simulink model "Mmc_GFL_template"  (R2024b)
settings: Solver=ode23t  StartTime=0.0  StopTime=.3  FixedStep=Ts_Power
undefined symbols (not defined in the file): Ch, Cm, Cmo, Fnom, fs, I_b, Ipp_b, kicir, kiout, kip, kpcir, kpout, kpp, L, L0, Nb_PM, R0, Rdis, Rh, Rm, SCR, SigmaM, Snom, Ts_Power, V_b, VDCm, VDCp, Vnom_AC, Vnom_PM, w_b, Zn
libraries: spsIGBTDiodeLib x48, spsSeriesRLCBranchLib x42, spsVoltageMeasurementLib x17, spsTriangleGeneratorLib x12, spsCurrentMeasurementLib x7, eePwmGeneratorMultilevel x7, slpidlib x6, spsFirstOrderFilterLib x4, spsabctodq0Lib x3, spsGroundLib x2, spsDCVoltageSourceLib x2, spsThreePhaseVIMeasurementLib x2
(part 2 of 3)

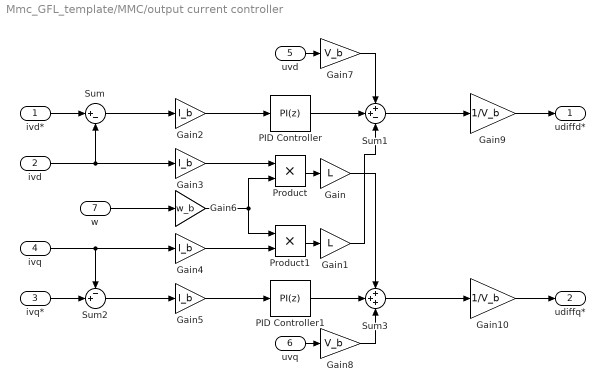
== system Mmc_GFL_template/MMC/output current controller ==
  ivd* : Inport
  ivd : Inport  Port=2
  ivq* : Inport  Port=3
  ivq : Inport  Port=4
  uvd : Inport  Port=5
  uvq : Inport  Port=6
  w : Inport  Port=7
  Gain : Gain  Gain=L
  Gain1 : Gain  Gain=L
  Gain10 : Gain  Gain=1/V_b
  Gain{2..5} (4 alike) : Gain  Gain=I_b
  Gain6 : Gain  Gain=w_b
  Gain7 : Gain  Gain=V_b
  Gain8 : Gain  Gain=V_b
  Gain9 : Gain  Gain=1/V_b
  PID Controller : slpidlib/PID Controller  Controller=PI  Form=Parallel  TimeDomain=Discrete-time  UseExternalTs=off  SampleTime=-1  IntegratorMethod=Forward Euler  FilterMethod=Forward Euler  ControllerParametersSource=internal  P=kpout  I=kiout  UseKiTs=off  D=0  UseExternalDerivativeSource=off  N=100  UseFilter=on  TunerSelectOption=Transfer Function Based (PID Tuner App)  InitialConditionSource=internal  InitialConditionForIntegrator=0  InitialConditionForFilter=0  DifferentiatorICPrevScaledInput=0  ExternalReset=none  TrackingMode=off  Kt=1  LimitOutput=off  SatLimitsSource=internal  UpperSaturationLimit=Vnom_AC  LowerSaturationLimit=-Vnom_AC  LinearizeAsGain=on  AntiWindupMode=clamping  Kb=1  LimitIntegrator=off  UpperIntegratorSaturationLimit=inf  LowerIntegratorSaturationLimit=-inf  POutMin=[]  POutMax=[]  IOutMin=[]  IOutMax=[]  DOutMin=[]  DOutMax=[]  NOutMin=[]  NOutMax=[]  SumOutMin=[]  SumOutMax=[]  SaturationOutMin=[]  SaturationOutMax=[]  PParamMin=[]  PParamMax=[]  IParamMin=[]  IParamMax=[]  DParamMin=[]  DParamMax=[]  NParamMin=[]  NParamMax=[]  KbParamMin=[]  KbParamMax=[]  KtParamMin=[]  KtParamMax=[]  KbOutMin=[]  KbOutMax=[]  KtOutMin=[]  KtOutMax=[]  IntegratorOutMin=[]  IntegratorOutMax=[]  FilterOutMin=[]  FilterOutMax=[]  SumI1OutMin=[]  SumI1OutMax=[]  SumI2OutMin=[]  SumI2OutMax=[]  SumI3OutMin=[]  SumI3OutMax=[]  SumI4OutMin=[]  SumI4OutMax=[]  SumDOutMin=[]  SumDOutMax=[]  DifferentiatorOutMin=[]  DifferentiatorOutMax=[]  FilterDiffOutCoefMin=[]  FilterDiffOutCoefMax=[]  ReciprocalOutMin=[]  ReciprocalOutMax=[]  SumDenOutMin=[]  SumDenOutMax=[]  SumNumOutMin=[]  SumNumOutMax=[]  DivideOutMin=[]  DivideOutMax=[]  UdiffTsProdOutMin=[]  UdiffTsProdOutMax=[]  NTsProdOutMin=[]  NTsProdOutMax=[]  UintegralTsProdOutMin=[]  UintegralTsProdOutMax=[]  UngainTsProdOutMin=[]  UngainTsProdOutMax=[]  ClampingZeroOutDataTypeStr=Inherit: Inherit via back propagation  ClampingZeroOutMin=[]  ClampingZeroOutMax=[]  FilterDenConstantOutDataTypeStr=Inherit: Inherit via back propagation  FilterDenConstantOutMin=[]  FilterDenConstantOutMax=[]  PCopyOutDataTypeStr=Inherit: Inherit via back propagation  PCopyOutMin=[]  PCopyOutMax=[]  NCopyOutDataTypeStr=Inherit: Inherit via back propagation  NCopyOutMin=[]  NCopyOutMax=[]  IntegratorContinuousStateAttributes=''  IntegratorStateMustResolveToSignalObject=off  IntegratorRTWStateStorageClass=Auto  FilterContinuousStateAttributes=''  FilterStateMustResolveToSignalObject=off  FilterRTWStateStorageClass=Auto  ParallelPVariant=InternalParameters  IdealPVariant=Disabled  IVariant=InternalParameters  DVariant=Disabled  IntegratorVariant=Discrete  SatVariant=Disabled  AWVariant=Passthrough  PCopyVariant=Disabled  TRVariant=Disabled  FdbkBlocksVariant=Forward  IdealPFdbkVariant=Disabled  SatFdbkVariant=Disabled  DerivativeFilterVariant=Disabled  NVariant=Disabled  NCopyVariant=Disabled_SignalSpec  FilterICVariant=Disabled  IntegratorICVariant=InternalICs  ExternalResetVariant=Disabled  TRSumVariant=Passthrough  SumFdbkVariant=Disabled  SumVariant=Sum_PI  TsampFilterVariant=InternalTs  TsampNgainVariant=Passthrough  TsampIntegralVariant=Disabled_SignalSpec  ExternalSaturationOutDataTypeStr=Inherit: Same as second input  DerivativeSourceVariant=Disabled  PreIntVariant=InternalPreInt
  PID Controller1 : slpidlib/PID Controller  Controller=PI  Form=Parallel  TimeDomain=Discrete-time  UseExternalTs=off  SampleTime=-1  IntegratorMethod=Forward Euler  FilterMethod=Forward Euler  ControllerParametersSource=internal  P=kpout  I=kiout  UseKiTs=off  D=0  UseExternalDerivativeSource=off  N=100  UseFilter=on  TunerSelectOption=Transfer Function Based (PID Tuner App)  InitialConditionSource=internal  InitialConditionForIntegrator=0  InitialConditionForFilter=0  DifferentiatorICPrevScaledInput=0  ExternalReset=none  TrackingMode=off  Kt=1  LimitOutput=off  SatLimitsSource=internal  UpperSaturationLimit=Vnom_AC  LowerSaturationLimit=-Vnom_AC  LinearizeAsGain=on  AntiWindupMode=clamping  Kb=1  LimitIntegrator=off  UpperIntegratorSaturationLimit=inf  LowerIntegratorSaturationLimit=-inf  POutMin=[]  POutMax=[]  IOutMin=[]  IOutMax=[]  DOutMin=[]  DOutMax=[]  NOutMin=[]  NOutMax=[]  SumOutMin=[]  SumOutMax=[]  SaturationOutMin=[]  SaturationOutMax=[]  PParamMin=[]  PParamMax=[]  IParamMin=[]  IParamMax=[]  DParamMin=[]  DParamMax=[]  NParamMin=[]  NParamMax=[]  KbParamMin=[]  KbParamMax=[]  KtParamMin=[]  KtParamMax=[]  KbOutMin=[]  KbOutMax=[]  KtOutMin=[]  KtOutMax=[]  IntegratorOutMin=[]  IntegratorOutMax=[]  FilterOutMin=[]  FilterOutMax=[]  SumI1OutMin=[]  SumI1OutMax=[]  SumI2OutMin=[]  SumI2OutMax=[]  SumI3OutMin=[]  SumI3OutMax=[]  SumI4OutMin=[]  SumI4OutMax=[]  SumDOutMin=[]  SumDOutMax=[]  DifferentiatorOutMin=[]  DifferentiatorOutMax=[]  FilterDiffOutCoefMin=[]  FilterDiffOutCoefMax=[]  ReciprocalOutMin=[]  ReciprocalOutMax=[]  SumDenOutMin=[]  SumDenOutMax=[]  SumNumOutMin=[]  SumNumOutMax=[]  DivideOutMin=[]  DivideOutMax=[]  UdiffTsProdOutMin=[]  UdiffTsProdOutMax=[]  NTsProdOutMin=[]  NTsProdOutMax=[]  UintegralTsProdOutMin=[]  UintegralTsProdOutMax=[]  UngainTsProdOutMin=[]  UngainTsProdOutMax=[]  ClampingZeroOutDataTypeStr=Inherit: Inherit via back propagation  ClampingZeroOutMin=[]  ClampingZeroOutMax=[]  FilterDenConstantOutDataTypeStr=Inherit: Inherit via back propagation  FilterDenConstantOutMin=[]  FilterDenConstantOutMax=[]  PCopyOutDataTypeStr=Inherit: Inherit via back propagation  PCopyOutMin=[]  PCopyOutMax=[]  NCopyOutDataTypeStr=Inherit: Inherit via back propagation  NCopyOutMin=[]  NCopyOutMax=[]  IntegratorContinuousStateAttributes=''  IntegratorStateMustResolveToSignalObject=off  IntegratorRTWStateStorageClass=Auto  FilterContinuousStateAttributes=''  FilterStateMustResolveToSignalObject=off  FilterRTWStateStorageClass=Auto  ParallelPVariant=InternalParameters  IdealPVariant=Disabled  IVariant=InternalParameters  DVariant=Disabled  IntegratorVariant=Discrete  SatVariant=Disabled  AWVariant=Passthrough  PCopyVariant=Disabled  TRVariant=Disabled  FdbkBlocksVariant=Forward  IdealPFdbkVariant=Disabled  SatFdbkVariant=Disabled  DerivativeFilterVariant=Disabled  NVariant=Disabled  NCopyVariant=Disabled_SignalSpec  FilterICVariant=Disabled  IntegratorICVariant=InternalICs  ExternalResetVariant=Disabled  TRSumVariant=Passthrough  SumFdbkVariant=Disabled  SumVariant=Sum_PI  TsampFilterVariant=InternalTs  TsampNgainVariant=Passthrough  TsampIntegralVariant=Disabled_SignalSpec  ExternalSaturationOutDataTypeStr=Inherit: Same as second input  DerivativeSourceVariant=Disabled  PreIntVariant=InternalPreInt
  Product : Product
  Product1 : Product
  Sum : Sum  Inputs=|+-
  Sum1 : Sum  Inputs=++-
  Sum2 : Sum  Inputs=-+|
  Sum3 : Sum  Inputs=+++
  udiffd* : Outport
  udiffq* : Outport  Port=2
  wires:
  ivd*/1 -> Sum/1
  ivd/1 -> Gain3/1, Sum/2
  Sum/1 -> Gain2/1
  PID Controller/1 -> Sum1/2
  uvd/1 -> Gain7/1
  Sum1/1 -> Gain9/1
  Sum2/1 -> Gain5/1
  PID Controller1/1 -> Sum3/2
  ivq*/1 -> Sum2/2
  ivq/1 -> Sum2/1, Gain4/1
  uvq/1 -> Gain8/1
  Sum3/1 -> Gain10/1
  Product/1 -> Gain/1
  Product1/1 -> Gain1/1
  Gain3/1 -> Product/1
  Gain4/1 -> Product1/2
  Gain5/1 -> PID Controller1/1
  w/1 -> Gain6/1
  Gain6/1 -> Product/2, Product1/1
  Gain9/1 -> udiffd*/1
  Gain10/1 -> udiffq*/1
  Gain7/1 -> Sum1/1
  Gain8/1 -> Sum3/3
  Gain2/1 -> PID Controller/1
  Gain/1 -> Sum3/1
  Gain1/1 -> Sum1/3

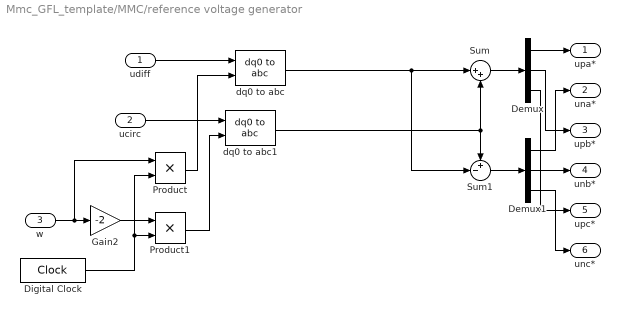
== system Mmc_GFL_template/MMC/reference voltage generator ==
  udiff : Inport
  ucirc : Inport  Port=2
  w : Inport  Port=3
  Demux : Demux  Outputs=3
  Demux1 : Demux  Outputs=3
  Digital Clock : DigitalClock  SampleTime=Ts_Power
  Gain2 : Gain  Gain=-2
  Product : Product
  Product1 : Product
  Sum : Sum  Inputs=|++
  Sum1 : Sum  Inputs=+-|
  dq0 to abc : spsdq0toabcLib/dq0 to abc  Alignment=90 degrees behind phase A axis
  dq0 to abc1 : spsdq0toabcLib/dq0 to abc  Alignment=90 degrees behind phase A axis
  upa* : Outport
  una* : Outport  Port=2
  upb* : Outport  Port=3
  unb* : Outport  Port=4
  upc* : Outport  Port=5
  unc* : Outport  Port=6
  wires:
  Product/1 -> dq0 to abc/2
  udiff/1 -> dq0 to abc/1
  ucirc/1 -> dq0 to abc1/1
  Digital Clock/1 -> Product/2, Product1/2
  Gain2/1 -> Product1/1
  Product1/1 -> dq0 to abc1/2
  w/1 -> Product/1, Gain2/1
  Demux/1 -> upa*/1
  Demux/2 -> upb*/1
  Demux/3 -> upc*/1
  Demux1/1 -> una*/1
  Demux1/2 -> unb*/1
  Demux1/3 -> unc*/1
  Sum/1 -> Demux/1
  Sum1/1 -> Demux1/1
  dq0 to abc1/1 -> Sum/2, Sum1/1
  dq0 to abc/1 -> Sum1/2, Sum/1

== system Mmc_GFL_template/MMC/Full-bridge/HBua1 ==
  gates : Inport
  Ch : spsSeriesRLCBranchLib/Series RLC Branch  LConnTagsString=__new0  RConnTagsString=__new0  BranchType=RC  Resistance=Rh(2,1)  Inductance=1e-3  SetiL0=off  InitialCurrent=0  Capacitance=Ch(2,1)  Setx0=off  InitialVoltage=750  Measurements=None
  Cm : spsSeriesRLCBranchLib/Series RLC Branch  LConnTagsString=__new0  RConnTagsString=__new0  BranchType=RC  Resistance=Rm(2,1)  Inductance=1e-3  SetiL0=off  InitialCurrent=0  Capacitance=Cmo(2,1)  Setx0=on  InitialVoltage=150  Measurements=None
  Demux1 : Demux
  IGBT/Diode{,1..3} (4 alike) : spsIGBTDiodeLib/IGBT//Diode  Ron=Ron  Rs=Rs  Cs=Cs  Measurements=off
  Rdis : spsSeriesRLCBranchLib/Series RLC Branch  LConnTagsString=__new0  RConnTagsString=__new0  BranchType=R  Resistance=Rdis(2,1)  Inductance=1e-3  SetiL0=off  InitialCurrent=0  Capacitance=Cm  Setx0=off  InitialVoltage=750  Measurements=None
  VA : PMIOPort  Side=Left
  VB : PMIOPort  Port=2  Side=Left
  DC+ : PMIOPort  Port=3  Side=Right
  DC- : PMIOPort  Port=4  Side=Right
  wires:
  gates/1 -> Demux1/1
  Demux1/4 -> IGBT/Diode3/1
  Demux1/3 -> IGBT/Diode2/1
  Demux1/2 -> IGBT/Diode1/1
  Demux1/1 -> IGBT/Diode/1
  connections:
  IGBT/Diode3/LConn1 -- VB/RConn1 -- IGBT/Diode2/RConn1
  Ch/LConn1 -- Rdis/LConn1 -- DC+/RConn1 -- IGBT/Diode/LConn1 -- IGBT/Diode2/LConn1 -- Cm/LConn1
  IGBT/Diode/RConn1 -- VA/RConn1 -- IGBT/Diode1/LConn1
  Ch/RConn1 -- DC-/RConn1 -- Rdis/RConn1 -- Cm/RConn1 -- IGBT/Diode3/RConn1 -- IGBT/Diode1/RConn1

== system Mmc_GFL_template/MMC/Full-bridge/HBua2 ==
  gates : Inport
  Ch : spsSeriesRLCBranchLib/Series RLC Branch  LConnTagsString=__new0  RConnTagsString=__new0  BranchType=RC  Resistance=Rh(2,1)  Inductance=1e-3  SetiL0=off  InitialCurrent=0  Capacitance=Ch(2,1)  Setx0=off  InitialVoltage=750  Measurements=None
  Cm : spsSeriesRLCBranchLib/Series RLC Branch  LConnTagsString=__new0  RConnTagsString=__new0  BranchType=RC  Resistance=Rm(2,1)  Inductance=1e-3  SetiL0=off  InitialCurrent=0  Capacitance=Cmo(2,1)  Setx0=on  InitialVoltage=150  Measurements=None
  Demux1 : Demux
  IGBT/Diode{,1..3} (4 alike) : spsIGBTDiodeLib/IGBT//Diode  Ron=Ron  Rs=Rs  Cs=Cs  Measurements=off
  Rdis : spsSeriesRLCBranchLib/Series RLC Branch  LConnTagsString=__new0  RConnTagsString=__new0  BranchType=R  Resistance=Rdis(2,1)  Inductance=1e-3  SetiL0=off  InitialCurrent=0  Capacitance=Cm  Setx0=off  InitialVoltage=750  Measurements=None
  VA : PMIOPort  Side=Left
  VB : PMIOPort  Port=2  Side=Left
  DC+ : PMIOPort  Port=3  Side=Right
  DC- : PMIOPort  Port=4  Side=Right
  wires:
  gates/1 -> Demux1/1
  Demux1/4 -> IGBT/Diode3/1
  Demux1/3 -> IGBT/Diode2/1
  Demux1/2 -> IGBT/Diode1/1
  Demux1/1 -> IGBT/Diode/1
  connections:
  IGBT/Diode3/LConn1 -- VB/RConn1 -- IGBT/Diode2/RConn1
  Ch/LConn1 -- Rdis/LConn1 -- DC+/RConn1 -- IGBT/Diode/LConn1 -- IGBT/Diode2/LConn1 -- Cm/LConn1
  IGBT/Diode/RConn1 -- VA/RConn1 -- IGBT/Diode1/LConn1
  Ch/RConn1 -- DC-/RConn1 -- Rdis/RConn1 -- Cm/RConn1 -- IGBT/Diode3/RConn1 -- IGBT/Diode1/RConn1

== system Mmc_GFL_template/MMC/Full-bridge 1/HBua1 ==
  gates : Inport
  Ch : spsSeriesRLCBranchLib/Series RLC Branch  LConnTagsString=__new0  RConnTagsString=__new0  BranchType=RC  Resistance=Rh(2,1)  Inductance=1e-3  SetiL0=off  InitialCurrent=0  Capacitance=Ch(2,1)  Setx0=off  InitialVoltage=750  Measurements=None
  Cm : spsSeriesRLCBranchLib/Series RLC Branch  LConnTagsString=__new0  RConnTagsString=__new0  BranchType=RC  Resistance=Rm(2,1)  Inductance=1e-3  SetiL0=off  InitialCurrent=0  Capacitance=Cmo(2,1)  Setx0=on  InitialVoltage=150  Measurements=None
  Demux1 : Demux
  IGBT/Diode{,1..3} (4 alike) : spsIGBTDiodeLib/IGBT//Diode  Ron=Ron  Rs=Rs  Cs=Cs  Measurements=off
  Rdis : spsSeriesRLCBranchLib/Series RLC Branch  LConnTagsString=__new0  RConnTagsString=__new0  BranchType=R  Resistance=Rdis(2,1)  Inductance=1e-3  SetiL0=off  InitialCurrent=0  Capacitance=Cm  Setx0=off  InitialVoltage=750  Measurements=None
  VA : PMIOPort  Side=Left
  VB : PMIOPort  Port=2  Side=Left
  DC+ : PMIOPort  Port=3  Side=Right
  DC- : PMIOPort  Port=4  Side=Right
  wires:
  gates/1 -> Demux1/1
  Demux1/4 -> IGBT/Diode3/1
  Demux1/3 -> IGBT/Diode2/1
  Demux1/2 -> IGBT/Diode1/1
  Demux1/1 -> IGBT/Diode/1
  connections:
  IGBT/Diode3/LConn1 -- VB/RConn1 -- IGBT/Diode2/RConn1
  Ch/LConn1 -- Rdis/LConn1 -- DC+/RConn1 -- IGBT/Diode/LConn1 -- IGBT/Diode2/LConn1 -- Cm/LConn1
  IGBT/Diode/RConn1 -- VA/RConn1 -- IGBT/Diode1/LConn1
  Ch/RConn1 -- DC-/RConn1 -- Rdis/RConn1 -- Cm/RConn1 -- IGBT/Diode3/RConn1 -- IGBT/Diode1/RConn1

== system Mmc_GFL_template/MMC/Full-bridge 1/HBua2 ==
  gates : Inport
  Ch : spsSeriesRLCBranchLib/Series RLC Branch  LConnTagsString=__new0  RConnTagsString=__new0  BranchType=RC  Resistance=Rh(2,1)  Inductance=1e-3  SetiL0=off  InitialCurrent=0  Capacitance=Ch(2,1)  Setx0=off  InitialVoltage=750  Measurements=None
  Cm : spsSeriesRLCBranchLib/Series RLC Branch  LConnTagsString=__new0  RConnTagsString=__new0  BranchType=RC  Resistance=Rm(2,1)  Inductance=1e-3  SetiL0=off  InitialCurrent=0  Capacitance=Cmo(2,1)  Setx0=on  InitialVoltage=150  Measurements=None
  Demux1 : Demux
  IGBT/Diode{,1..3} (4 alike) : spsIGBTDiodeLib/IGBT//Diode  Ron=Ron  Rs=Rs  Cs=Cs  Measurements=off
  Rdis : spsSeriesRLCBranchLib/Series RLC Branch  LConnTagsString=__new0  RConnTagsString=__new0  BranchType=R  Resistance=Rdis(2,1)  Inductance=1e-3  SetiL0=off  InitialCurrent=0  Capacitance=Cm  Setx0=off  InitialVoltage=750  Measurements=None
  VA : PMIOPort  Side=Left
  VB : PMIOPort  Port=2  Side=Left
  DC+ : PMIOPort  Port=3  Side=Right
  DC- : PMIOPort  Port=4  Side=Right
  wires:
  gates/1 -> Demux1/1
  Demux1/4 -> IGBT/Diode3/1
  Demux1/3 -> IGBT/Diode2/1
  Demux1/2 -> IGBT/Diode1/1
  Demux1/1 -> IGBT/Diode/1
  connections:
  IGBT/Diode3/LConn1 -- VB/RConn1 -- IGBT/Diode2/RConn1
  Ch/LConn1 -- Rdis/LConn1 -- DC+/RConn1 -- IGBT/Diode/LConn1 -- IGBT/Diode2/LConn1 -- Cm/LConn1
  IGBT/Diode/RConn1 -- VA/RConn1 -- IGBT/Diode1/LConn1
  Ch/RConn1 -- DC-/RConn1 -- Rdis/RConn1 -- Cm/RConn1 -- IGBT/Diode3/RConn1 -- IGBT/Diode1/RConn1

== system Mmc_GFL_template/MMC/Full-bridge 2/HBua1 ==
  gates : Inport
  Ch : spsSeriesRLCBranchLib/Series RLC Branch  LConnTagsString=__new0  RConnTagsString=__new0  BranchType=RC  Resistance=Rh(2,1)  Inductance=1e-3  SetiL0=off  InitialCurrent=0  Capacitance=Ch(2,1)  Setx0=off  InitialVoltage=750  Measurements=None
  Cm : spsSeriesRLCBranchLib/Series RLC Branch  LConnTagsString=__new0  RConnTagsString=__new0  BranchType=RC  Resistance=Rm(2,1)  Inductance=1e-3  SetiL0=off  InitialCurrent=0  Capacitance=Cmo(2,1)  Setx0=on  InitialVoltage=150  Measurements=None
  Demux1 : Demux
  IGBT/Diode{,1..3} (4 alike) : spsIGBTDiodeLib/IGBT//Diode  Ron=Ron  Rs=Rs  Cs=Cs  Measurements=off
  Rdis : spsSeriesRLCBranchLib/Series RLC Branch  LConnTagsString=__new0  RConnTagsString=__new0  BranchType=R  Resistance=Rdis(2,1)  Inductance=1e-3  SetiL0=off  InitialCurrent=0  Capacitance=Cm  Setx0=off  InitialVoltage=750  Measurements=None
  VA : PMIOPort  Side=Left
  VB : PMIOPort  Port=2  Side=Left
  DC+ : PMIOPort  Port=3  Side=Right
  DC- : PMIOPort  Port=4  Side=Right
  wires:
  gates/1 -> Demux1/1
  Demux1/4 -> IGBT/Diode3/1
  Demux1/3 -> IGBT/Diode2/1
  Demux1/2 -> IGBT/Diode1/1
  Demux1/1 -> IGBT/Diode/1
  connections:
  IGBT/Diode3/LConn1 -- VB/RConn1 -- IGBT/Diode2/RConn1
  Ch/LConn1 -- Rdis/LConn1 -- DC+/RConn1 -- IGBT/Diode/LConn1 -- IGBT/Diode2/LConn1 -- Cm/LConn1
  IGBT/Diode/RConn1 -- VA/RConn1 -- IGBT/Diode1/LConn1
  Ch/RConn1 -- DC-/RConn1 -- Rdis/RConn1 -- Cm/RConn1 -- IGBT/Diode3/RConn1 -- IGBT/Diode1/RConn1

== system Mmc_GFL_template/MMC/Full-bridge 2/HBua2 ==
  gates : Inport
  Ch : spsSeriesRLCBranchLib/Series RLC Branch  LConnTagsString=__new0  RConnTagsString=__new0  BranchType=RC  Resistance=Rh(2,1)  Inductance=1e-3  SetiL0=off  InitialCurrent=0  Capacitance=Ch(2,1)  Setx0=off  InitialVoltage=750  Measurements=None
  Cm : spsSeriesRLCBranchLib/Series RLC Branch  LConnTagsString=__new0  RConnTagsString=__new0  BranchType=RC  Resistance=Rm(2,1)  Inductance=1e-3  SetiL0=off  InitialCurrent=0  Capacitance=Cmo(2,1)  Setx0=on  InitialVoltage=150  Measurements=None
  Demux1 : Demux
  IGBT/Diode{,1..3} (4 alike) : spsIGBTDiodeLib/IGBT//Diode  Ron=Ron  Rs=Rs  Cs=Cs  Measurements=off
  Rdis : spsSeriesRLCBranchLib/Series RLC Branch  LConnTagsString=__new0  RConnTagsString=__new0  BranchType=R  Resistance=Rdis(2,1)  Inductance=1e-3  SetiL0=off  InitialCurrent=0  Capacitance=Cm  Setx0=off  InitialVoltage=750  Measurements=None
  VA : PMIOPort  Side=Left
  VB : PMIOPort  Port=2  Side=Left
  DC+ : PMIOPort  Port=3  Side=Right
  DC- : PMIOPort  Port=4  Side=Right
  wires:
  gates/1 -> Demux1/1
  Demux1/4 -> IGBT/Diode3/1
  Demux1/3 -> IGBT/Diode2/1
  Demux1/2 -> IGBT/Diode1/1
  Demux1/1 -> IGBT/Diode/1
  connections:
  IGBT/Diode3/LConn1 -- VB/RConn1 -- IGBT/Diode2/RConn1
  Ch/LConn1 -- Rdis/LConn1 -- DC+/RConn1 -- IGBT/Diode/LConn1 -- IGBT/Diode2/LConn1 -- Cm/LConn1
  IGBT/Diode/RConn1 -- VA/RConn1 -- IGBT/Diode1/LConn1
  Ch/RConn1 -- DC-/RConn1 -- Rdis/RConn1 -- Cm/RConn1 -- IGBT/Diode3/RConn1 -- IGBT/Diode1/RConn1

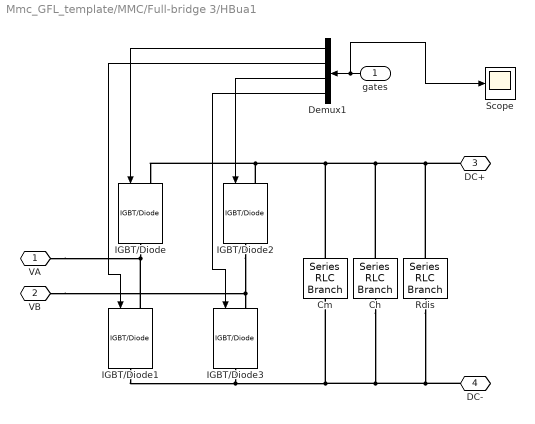
== system Mmc_GFL_template/MMC/Full-bridge 3/HBua1 ==
  gates : Inport
  Ch : spsSeriesRLCBranchLib/Series RLC Branch  LConnTagsString=__new0  RConnTagsString=__new0  BranchType=RC  Resistance=Rh(2,1)  Inductance=1e-3  SetiL0=off  InitialCurrent=0  Capacitance=Ch(2,1)  Setx0=off  InitialVoltage=750  Measurements=None
  Cm : spsSeriesRLCBranchLib/Series RLC Branch  LConnTagsString=__new0  RConnTagsString=__new0  BranchType=RC  Resistance=Rm(2,1)  Inductance=1e-3  SetiL0=off  InitialCurrent=0  Capacitance=Cmo(2,1)  Setx0=on  InitialVoltage=150  Measurements=None
  Demux1 : Demux
  IGBT/Diode{,1..3} (4 alike) : spsIGBTDiodeLib/IGBT//Diode  Ron=Ron  Rs=Rs  Cs=Cs  Measurements=off
  Rdis : spsSeriesRLCBranchLib/Series RLC Branch  LConnTagsString=__new0  RConnTagsString=__new0  BranchType=R  Resistance=Rdis(2,1)  Inductance=1e-3  SetiL0=off  InitialCurrent=0  Capacitance=Cm  Setx0=off  InitialVoltage=750  Measurements=None
  Scope : Scope
  VA : PMIOPort  Side=Left
  VB : PMIOPort  Port=2  Side=Left
  DC+ : PMIOPort  Port=3  Side=Right
  DC- : PMIOPort  Port=4  Side=Right
  wires:
  gates/1 -> Scope/1, Demux1/1
  Demux1/4 -> IGBT/Diode3/1
  Demux1/3 -> IGBT/Diode2/1
  Demux1/2 -> IGBT/Diode1/1
  Demux1/1 -> IGBT/Diode/1
  connections:
  IGBT/Diode3/LConn1 -- VB/RConn1 -- IGBT/Diode2/RConn1
  Ch/LConn1 -- Rdis/LConn1 -- DC+/RConn1 -- IGBT/Diode/LConn1 -- IGBT/Diode2/LConn1 -- Cm/LConn1
  IGBT/Diode/RConn1 -- VA/RConn1 -- IGBT/Diode1/LConn1
  Ch/RConn1 -- DC-/RConn1 -- Rdis/RConn1 -- Cm/RConn1 -- IGBT/Diode3/RConn1 -- IGBT/Diode1/RConn1

== system Mmc_GFL_template/MMC/Full-bridge 3/HBua2 ==
  gates : Inport
  Ch : spsSeriesRLCBranchLib/Series RLC Branch  LConnTagsString=__new0  RConnTagsString=__new0  BranchType=RC  Resistance=Rh(2,1)  Inductance=1e-3  SetiL0=off  InitialCurrent=0  Capacitance=Ch(2,1)  Setx0=off  InitialVoltage=750  Measurements=None
  Cm : spsSeriesRLCBranchLib/Series RLC Branch  LConnTagsString=__new0  RConnTagsString=__new0  BranchType=RC  Resistance=Rm(2,1)  Inductance=1e-3  SetiL0=off  InitialCurrent=0  Capacitance=Cmo(2,1)  Setx0=on  InitialVoltage=150  Measurements=None
  Demux1 : Demux
  IGBT/Diode{,1..3} (4 alike) : spsIGBTDiodeLib/IGBT//Diode  Ron=Ron  Rs=Rs  Cs=Cs  Measurements=off
  Rdis : spsSeriesRLCBranchLib/Series RLC Branch  LConnTagsString=__new0  RConnTagsString=__new0  BranchType=R  Resistance=Rdis(2,1)  Inductance=1e-3  SetiL0=off  InitialCurrent=0  Capacitance=Cm  Setx0=off  InitialVoltage=750  Measurements=None
  VA : PMIOPort  Side=Left
  VB : PMIOPort  Port=2  Side=Left
  DC+ : PMIOPort  Port=3  Side=Right
  DC- : PMIOPort  Port=4  Side=Right
  wires:
  gates/1 -> Demux1/1
  Demux1/4 -> IGBT/Diode3/1
  Demux1/3 -> IGBT/Diode2/1
  Demux1/2 -> IGBT/Diode1/1
  Demux1/1 -> IGBT/Diode/1
  connections:
  IGBT/Diode3/LConn1 -- VB/RConn1 -- IGBT/Diode2/RConn1
  Ch/LConn1 -- Rdis/LConn1 -- DC+/RConn1 -- IGBT/Diode/LConn1 -- IGBT/Diode2/LConn1 -- Cm/LConn1
  IGBT/Diode/RConn1 -- VA/RConn1 -- IGBT/Diode1/LConn1
  Ch/RConn1 -- DC-/RConn1 -- Rdis/RConn1 -- Cm/RConn1 -- IGBT/Diode3/RConn1 -- IGBT/Diode1/RConn1

== system Mmc_GFL_template/MMC/Full-bridge 4/HBua1 ==
  gates : Inport
  Ch : spsSeriesRLCBranchLib/Series RLC Branch  LConnTagsString=__new0  RConnTagsString=__new0  BranchType=RC  Resistance=Rh(2,1)  Inductance=1e-3  SetiL0=off  InitialCurrent=0  Capacitance=Ch(2,1)  Setx0=off  InitialVoltage=750  Measurements=None
  Cm : spsSeriesRLCBranchLib/Series RLC Branch  LConnTagsString=__new0  RConnTagsString=__new0  BranchType=RC  Resistance=Rm(2,1)  Inductance=1e-3  SetiL0=off  InitialCurrent=0  Capacitance=Cmo(2,1)  Setx0=on  InitialVoltage=150  Measurements=None
  Demux1 : Demux
  IGBT/Diode{,1..3} (4 alike) : spsIGBTDiodeLib/IGBT//Diode  Ron=Ron  Rs=Rs  Cs=Cs  Measurements=off
  Rdis : spsSeriesRLCBranchLib/Series RLC Branch  LConnTagsString=__new0  RConnTagsString=__new0  BranchType=R  Resistance=Rdis(2,1)  Inductance=1e-3  SetiL0=off  InitialCurrent=0  Capacitance=Cm  Setx0=off  InitialVoltage=750  Measurements=None
  VA : PMIOPort  Side=Left
  VB : PMIOPort  Port=2  Side=Left
  DC+ : PMIOPort  Port=3  Side=Right
  DC- : PMIOPort  Port=4  Side=Right
  wires:
  gates/1 -> Demux1/1
  Demux1/4 -> IGBT/Diode3/1
  Demux1/3 -> IGBT/Diode2/1
  Demux1/2 -> IGBT/Diode1/1
  Demux1/1 -> IGBT/Diode/1
  connections:
  IGBT/Diode3/LConn1 -- VB/RConn1 -- IGBT/Diode2/RConn1
  Ch/LConn1 -- Rdis/LConn1 -- DC+/RConn1 -- IGBT/Diode/LConn1 -- IGBT/Diode2/LConn1 -- Cm/LConn1
  IGBT/Diode/RConn1 -- VA/RConn1 -- IGBT/Diode1/LConn1
  Ch/RConn1 -- DC-/RConn1 -- Rdis/RConn1 -- Cm/RConn1 -- IGBT/Diode3/RConn1 -- IGBT/Diode1/RConn1

== system Mmc_GFL_template/MMC/Full-bridge 4/HBua2 ==
  gates : Inport
  Ch : spsSeriesRLCBranchLib/Series RLC Branch  LConnTagsString=__new0  RConnTagsString=__new0  BranchType=RC  Resistance=Rh(2,1)  Inductance=1e-3  SetiL0=off  InitialCurrent=0  Capacitance=Ch(2,1)  Setx0=off  InitialVoltage=750  Measurements=None
  Cm : spsSeriesRLCBranchLib/Series RLC Branch  LConnTagsString=__new0  RConnTagsString=__new0  BranchType=RC  Resistance=Rm(2,1)  Inductance=1e-3  SetiL0=off  InitialCurrent=0  Capacitance=Cmo(2,1)  Setx0=on  InitialVoltage=150  Measurements=None
  Demux1 : Demux
  IGBT/Diode{,1..3} (4 alike) : spsIGBTDiodeLib/IGBT//Diode  Ron=Ron  Rs=Rs  Cs=Cs  Measurements=off
  Rdis : spsSeriesRLCBranchLib/Series RLC Branch  LConnTagsString=__new0  RConnTagsString=__new0  BranchType=R  Resistance=Rdis(2,1)  Inductance=1e-3  SetiL0=off  InitialCurrent=0  Capacitance=Cm  Setx0=off  InitialVoltage=750  Measurements=None
  VA : PMIOPort  Side=Left
  VB : PMIOPort  Port=2  Side=Left
  DC+ : PMIOPort  Port=3  Side=Right
  DC- : PMIOPort  Port=4  Side=Right
  wires:
  gates/1 -> Demux1/1
  Demux1/4 -> IGBT/Diode3/1
  Demux1/3 -> IGBT/Diode2/1
  Demux1/2 -> IGBT/Diode1/1
  Demux1/1 -> IGBT/Diode/1
  connections:
  IGBT/Diode3/LConn1 -- VB/RConn1 -- IGBT/Diode2/RConn1
  Ch/LConn1 -- Rdis/LConn1 -- DC+/RConn1 -- IGBT/Diode/LConn1 -- IGBT/Diode2/LConn1 -- Cm/LConn1
  IGBT/Diode/RConn1 -- VA/RConn1 -- IGBT/Diode1/LConn1
  Ch/RConn1 -- DC-/RConn1 -- Rdis/RConn1 -- Cm/RConn1 -- IGBT/Diode3/RConn1 -- IGBT/Diode1/RConn1

== system Mmc_GFL_template/MMC/Full-bridge 5/HBua1 ==
  gates : Inport
  Ch : spsSeriesRLCBranchLib/Series RLC Branch  LConnTagsString=__new0  RConnTagsString=__new0  BranchType=RC  Resistance=Rh(2,1)  Inductance=1e-3  SetiL0=off  InitialCurrent=0  Capacitance=Ch(2,1)  Setx0=off  InitialVoltage=750  Measurements=None
  Cm : spsSeriesRLCBranchLib/Series RLC Branch  LConnTagsString=__new0  RConnTagsString=__new0  BranchType=RC  Resistance=Rm(2,1)  Inductance=1e-3  SetiL0=off  InitialCurrent=0  Capacitance=Cmo(2,1)  Setx0=on  InitialVoltage=150  Measurements=None
  Demux1 : Demux
  IGBT/Diode{,1..3} (4 alike) : spsIGBTDiodeLib/IGBT//Diode  Ron=Ron  Rs=Rs  Cs=Cs  Measurements=off
  Rdis : spsSeriesRLCBranchLib/Series RLC Branch  LConnTagsString=__new0  RConnTagsString=__new0  BranchType=R  Resistance=Rdis(2,1)  Inductance=1e-3  SetiL0=off  InitialCurrent=0  Capacitance=Cm  Setx0=off  InitialVoltage=750  Measurements=None
  VA : PMIOPort  Side=Left
  VB : PMIOPort  Port=2  Side=Left
  DC+ : PMIOPort  Port=3  Side=Right
  DC- : PMIOPort  Port=4  Side=Right
  wires:
  gates/1 -> Demux1/1
  Demux1/4 -> IGBT/Diode3/1
  Demux1/3 -> IGBT/Diode2/1
  Demux1/2 -> IGBT/Diode1/1
  Demux1/1 -> IGBT/Diode/1
  connections:
  IGBT/Diode3/LConn1 -- VB/RConn1 -- IGBT/Diode2/RConn1
  Ch/LConn1 -- Rdis/LConn1 -- DC+/RConn1 -- IGBT/Diode/LConn1 -- IGBT/Diode2/LConn1 -- Cm/LConn1
  IGBT/Diode/RConn1 -- VA/RConn1 -- IGBT/Diode1/LConn1
  Ch/RConn1 -- DC-/RConn1 -- Rdis/RConn1 -- Cm/RConn1 -- IGBT/Diode3/RConn1 -- IGBT/Diode1/RConn1

== system Mmc_GFL_template/MMC/Full-bridge 5/HBua2 ==
  gates : Inport
  Ch : spsSeriesRLCBranchLib/Series RLC Branch  LConnTagsString=__new0  RConnTagsString=__new0  BranchType=RC  Resistance=Rh(2,1)  Inductance=1e-3  SetiL0=off  InitialCurrent=0  Capacitance=Ch(2,1)  Setx0=off  InitialVoltage=750  Measurements=None
  Cm : spsSeriesRLCBranchLib/Series RLC Branch  LConnTagsString=__new0  RConnTagsString=__new0  BranchType=RC  Resistance=Rm(2,1)  Inductance=1e-3  SetiL0=off  InitialCurrent=0  Capacitance=Cmo(2,1)  Setx0=on  InitialVoltage=150  Measurements=None
  Demux1 : Demux
  IGBT/Diode{,1..3} (4 alike) : spsIGBTDiodeLib/IGBT//Diode  Ron=Ron  Rs=Rs  Cs=Cs  Measurements=off
  Rdis : spsSeriesRLCBranchLib/Series RLC Branch  LConnTagsString=__new0  RConnTagsString=__new0  BranchType=R  Resistance=Rdis(2,1)  Inductance=1e-3  SetiL0=off  InitialCurrent=0  Capacitance=Cm  Setx0=off  InitialVoltage=750  Measurements=None
  VA : PMIOPort  Side=Left
  VB : PMIOPort  Port=2  Side=Left
  DC+ : PMIOPort  Port=3  Side=Right
  DC- : PMIOPort  Port=4  Side=Right
  wires:
  gates/1 -> Demux1/1
  Demux1/4 -> IGBT/Diode3/1
  Demux1/3 -> IGBT/Diode2/1
  Demux1/2 -> IGBT/Diode1/1
  Demux1/1 -> IGBT/Diode/1
  connections:
  IGBT/Diode3/LConn1 -- VB/RConn1 -- IGBT/Diode2/RConn1
  Ch/LConn1 -- Rdis/LConn1 -- DC+/RConn1 -- IGBT/Diode/LConn1 -- IGBT/Diode2/LConn1 -- Cm/LConn1
  IGBT/Diode/RConn1 -- VA/RConn1 -- IGBT/Diode1/LConn1
  Ch/RConn1 -- DC-/RConn1 -- Rdis/RConn1 -- Cm/RConn1 -- IGBT/Diode3/RConn1 -- IGBT/Diode1/RConn1

== system Mmc_GFL_template/MMC/PS-PWM/PS-PWM lower a ==
  ref : Inport
  Gain : Gain  Gain=70
  Gain1 : Gain  Gain=70
  Logical Operator : Logic  Operator=NOT  AllPortsSameDT=off  OutDataTypeStr=boolean
  Logical Operator1 : Logic  Operator=NOT  AllPortsSameDT=off  OutDataTypeStr=boolean
  Mux : Mux
  Relational Operator : RelationalOperator  OutDataTypeStr=boolean  RndMeth=Simplest  InputSameDT=off
  Relational Operator1 : RelationalOperator  OutDataTypeStr=boolean  RndMeth=Simplest  InputSameDT=off
  Triangle Generator : spsTriangleGeneratorLib/Triangle Generator  Freq=1e3  Phase=0  Ts=Ts_Power
  Triangle Generator1 : spsTriangleGeneratorLib/Triangle Generator  Freq=1e3  Phase=pi/(4)  Ts=Ts_Power
  Ppa : Outport
  wires:
  Logical Operator/1 -> Mux/2
  ref/1 -> Relational Operator1/1, Relational Operator/1
  Relational Operator/1 -> Mux/1, Logical Operator/1
  Relational Operator1/1 -> Logical Operator1/1, Mux/3
  Triangle Generator/1 -> Gain/1
  Triangle Generator1/1 -> Gain1/1
  Mux/1 -> Ppa/1
  Logical Operator1/1 -> Mux/4
  Gain1/1 -> Relational Operator1/2
  Gain/1 -> Relational Operator/2

== system Mmc_GFL_template/MMC/PS-PWM/PS-PWM lower b ==
  ref : Inport
  Gain : Gain  Gain=70
  Gain1 : Gain  Gain=70
  Logical Operator : Logic  Operator=NOT  AllPortsSameDT=off  OutDataTypeStr=boolean
  Logical Operator1 : Logic  Operator=NOT  AllPortsSameDT=off  OutDataTypeStr=boolean
  Mux : Mux
  Relational Operator : RelationalOperator  OutDataTypeStr=boolean  RndMeth=Simplest  InputSameDT=off
  Relational Operator1 : RelationalOperator  OutDataTypeStr=boolean  RndMeth=Simplest  InputSameDT=off
  Triangle Generator : spsTriangleGeneratorLib/Triangle Generator  Freq=1e3  Phase=0  Ts=Ts_Power
  Triangle Generator1 : spsTriangleGeneratorLib/Triangle Generator  Freq=1e3  Phase=pi/(4)  Ts=Ts_Power
  Ppa : Outport
  wires:
  Logical Operator/1 -> Mux/2
  ref/1 -> Relational Operator1/1, Relational Operator/1
  Relational Operator/1 -> Mux/1, Logical Operator/1
  Relational Operator1/1 -> Logical Operator1/1, Mux/3
  Triangle Generator/1 -> Gain/1
  Triangle Generator1/1 -> Gain1/1
  Mux/1 -> Ppa/1
  Logical Operator1/1 -> Mux/4
  Gain/1 -> Relational Operator/2
  Gain1/1 -> Relational Operator1/2

== system Mmc_GFL_template/MMC/PS-PWM/PS-PWM lower c ==
  ref : Inport
  Gain : Gain  Gain=70
  Gain1 : Gain  Gain=70
  Logical Operator : Logic  Operator=NOT  AllPortsSameDT=off  OutDataTypeStr=boolean
  Logical Operator1 : Logic  Operator=NOT  AllPortsSameDT=off  OutDataTypeStr=boolean
  Mux : Mux
  Relational Operator : RelationalOperator  OutDataTypeStr=boolean  RndMeth=Simplest  InputSameDT=off
  Relational Operator1 : RelationalOperator  OutDataTypeStr=boolean  RndMeth=Simplest  InputSameDT=off
  Triangle Generator : spsTriangleGeneratorLib/Triangle Generator  Freq=1e3  Phase=0  Ts=Ts_Power
  Triangle Generator1 : spsTriangleGeneratorLib/Triangle Generator  Freq=1e3  Phase=pi/(4)  Ts=Ts_Power
  Ppa : Outport
  wires:
  Logical Operator/1 -> Mux/2
  ref/1 -> Relational Operator1/1, Relational Operator/1
  Relational Operator/1 -> Mux/1, Logical Operator/1
  Relational Operator1/1 -> Logical Operator1/1, Mux/3
  Triangle Generator/1 -> Gain/1
  Triangle Generator1/1 -> Gain1/1
  Mux/1 -> Ppa/1
  Logical Operator1/1 -> Mux/4
  Gain/1 -> Relational Operator/2
  Gain1/1 -> Relational Operator1/2

== system Mmc_GFL_template/MMC/PS-PWM/PS-PWM upper a ==
  ref : Inport
  Gain : Gain  Gain=70
  Gain1 : Gain  Gain=70
  Logical Operator : Logic  Operator=NOT  AllPortsSameDT=off  OutDataTypeStr=boolean
  Logical Operator1 : Logic  Operator=NOT  AllPortsSameDT=off  OutDataTypeStr=boolean
  Mux : Mux
  Relational Operator : RelationalOperator  OutDataTypeStr=boolean  RndMeth=Simplest  InputSameDT=off
  Relational Operator1 : RelationalOperator  OutDataTypeStr=boolean  RndMeth=Simplest  InputSameDT=off
  Scope : Scope
  Triangle Generator : spsTriangleGeneratorLib/Triangle Generator  Freq=1e3  Phase=0  Ts=Ts_Power
  Triangle Generator1 : spsTriangleGeneratorLib/Triangle Generator  Freq=1e3  Phase=pi/(4)  Ts=Ts_Power
  Ppa : Outport
  wires:
  Triangle Generator1/1 -> Gain1/1
  Triangle Generator/1 -> Gain/1
  ref/1 -> Scope/1, Relational Operator1/1, Relational Operator/1
  Mux/1 -> Ppa/1
  Relational Operator/1 -> Mux/1, Logical Operator/1
  Relational Operator1/1 -> Logical Operator1/1, Mux/3
  Logical Operator/1 -> Mux/2
  Logical Operator1/1 -> Mux/4
  Gain/1 -> Relational Operator/2
  Gain1/1 -> Relational Operator1/2

== system Mmc_GFL_template/MMC/PS-PWM/PS-PWM upper b ==
  ref : Inport
  Gain : Gain  Gain=70
  Gain1 : Gain  Gain=70
  Logical Operator : Logic  Operator=NOT  AllPortsSameDT=off  OutDataTypeStr=boolean
  Logical Operator1 : Logic  Operator=NOT  AllPortsSameDT=off  OutDataTypeStr=boolean
  Mux : Mux
  Relational Operator : RelationalOperator  OutDataTypeStr=boolean  RndMeth=Simplest  InputSameDT=off
  Relational Operator1 : RelationalOperator  OutDataTypeStr=boolean  RndMeth=Simplest  InputSameDT=off
  Triangle Generator : spsTriangleGeneratorLib/Triangle Generator  Freq=1e3  Phase=0  Ts=Ts_Power
  Triangle Generator1 : spsTriangleGeneratorLib/Triangle Generator  Freq=1e3  Phase=pi/(4)  Ts=Ts_Power
  Ppa : Outport
  wires:
  Triangle Generator1/1 -> Gain1/1
  Triangle Generator/1 -> Gain/1
  ref/1 -> Relational Operator1/1, Relational Operator/1
  Mux/1 -> Ppa/1
  Relational Operator/1 -> Mux/1, Logical Operator/1
  Relational Operator1/1 -> Logical Operator1/1, Mux/3
  Logical Operator/1 -> Mux/2
  Logical Operator1/1 -> Mux/4
  Gain/1 -> Relational Operator/2
  Gain1/1 -> Relational Operator1/2

== system Mmc_GFL_template/MMC/PS-PWM/PS-PWM upper c ==
  ref : Inport
  Gain : Gain  Gain=70
  Gain1 : Gain  Gain=70
  Logical Operator : Logic  Operator=NOT  AllPortsSameDT=off  OutDataTypeStr=boolean
  Logical Operator1 : Logic  Operator=NOT  AllPortsSameDT=off  OutDataTypeStr=boolean
  Mux : Mux
  Relational Operator : RelationalOperator  OutDataTypeStr=boolean  RndMeth=Simplest  InputSameDT=off
  Relational Operator1 : RelationalOperator  OutDataTypeStr=boolean  RndMeth=Simplest  InputSameDT=off
  Triangle Generator : spsTriangleGeneratorLib/Triangle Generator  Freq=1e3  Phase=0  Ts=Ts_Power
  Triangle Generator1 : spsTriangleGeneratorLib/Triangle Generator  Freq=1e3  Phase=pi/(4)  Ts=Ts_Power
  Ppa : Outport
  wires:
  Triangle Generator1/1 -> Gain1/1
  Triangle Generator/1 -> Gain/1
  ref/1 -> Relational Operator1/1, Relational Operator/1
  Mux/1 -> Ppa/1
  Relational Operator/1 -> Mux/1, Logical Operator/1
  Relational Operator1/1 -> Logical Operator1/1, Mux/3
  Logical Operator/1 -> Mux/2
  Logical Operator1/1 -> Mux/4
  Gain/1 -> Relational Operator/2
  Gain1/1 -> Relational Operator1/2

== system Mmc_GFL_template/MMC/modulation/Sorting na ==
  note: A secrect, unintelligible, confusing and insrutable function with \if inside \for inside \if inside \if inside \if
  Usm : Inport
  N : Inport  Port=2
  Iarm : Inport  Port=3
  Constant : Constant  Value=SigmaM
  Logical Operator : Logic  Operator=NOT  AllPortsSameDT=off  OutDataTypeStr=float('double')
  MATLAB Function : MATLAB Function  TreatAsAtomicUnit=on
  MATLAB Function1 : MATLAB Function  TreatAsAtomicUnit=on
  Memory : Memory  InitialCondition=logical(zeros(Nb_PM, 1))  InheritSampleTime=on
  Mux : Mux  Inputs=2
  firing : Outport
  wires:
  MATLAB Function1/1(y) -> firing/1
  Logical Operator/1 -> Mux/2
  MATLAB Function/1(Ons_next) -> Mux/1, Logical Operator/1, Memory/1
  Mux/1 -> MATLAB Function1/1(u)
  Usm/1 -> MATLAB Function/1(Usm)
  Constant/1 -> MATLAB Function/3(Sigmam)
  N/1 -> MATLAB Function/2(N)
  Memory/1 -> MATLAB Function/5(Ons)
  Iarm/1 -> MATLAB Function/4(Iarm)

== system Mmc_GFL_template/MMC/modulation/Sorting nb ==
  note: A secrect, unintelligible, confusing and insrutable function with \if inside \for inside \if inside \if inside \if
  Usm : Inport
  N : Inport  Port=2
  Iarm : Inport  Port=3
  Constant : Constant  Value=SigmaM
  Logical Operator : Logic  Operator=NOT  AllPortsSameDT=off  OutDataTypeStr=float('double')
  MATLAB Function : MATLAB Function  TreatAsAtomicUnit=on
  MATLAB Function1 : MATLAB Function  TreatAsAtomicUnit=on
  Memory : Memory  InitialCondition=logical(zeros(Nb_PM, 1))  InheritSampleTime=on
  Mux : Mux  Inputs=2
  firing : Outport
  wires:
  MATLAB Function1/1(y) -> firing/1
  Logical Operator/1 -> Mux/2
  MATLAB Function/1(Ons_next) -> Mux/1, Logical Operator/1, Memory/1
  Mux/1 -> MATLAB Function1/1(u)
  Usm/1 -> MATLAB Function/1(Usm)
  Constant/1 -> MATLAB Function/3(Sigmam)
  N/1 -> MATLAB Function/2(N)
  Memory/1 -> MATLAB Function/5(Ons)
  Iarm/1 -> MATLAB Function/4(Iarm)

== system Mmc_GFL_template/MMC/modulation/Sorting nc ==
  note: A secrect, unintelligible, confusing and insrutable function with \if inside \for inside \if inside \if inside \if
  Usm : Inport
  N : Inport  Port=2
  Iarm : Inport  Port=3
  Constant : Constant  Value=SigmaM
  Logical Operator : Logic  Operator=NOT  AllPortsSameDT=off  OutDataTypeStr=float('double')
  MATLAB Function : MATLAB Function  TreatAsAtomicUnit=on
  MATLAB Function1 : MATLAB Function  TreatAsAtomicUnit=on
  Memory : Memory  InitialCondition=logical(zeros(Nb_PM, 1))  InheritSampleTime=on
  Mux : Mux  Inputs=2
  firing : Outport
  wires:
  MATLAB Function1/1(y) -> firing/1
  Logical Operator/1 -> Mux/2
  MATLAB Function/1(Ons_next) -> Mux/1, Logical Operator/1, Memory/1
  Mux/1 -> MATLAB Function1/1(u)
  Usm/1 -> MATLAB Function/1(Usm)
  Constant/1 -> MATLAB Function/3(Sigmam)
  N/1 -> MATLAB Function/2(N)
  Memory/1 -> MATLAB Function/5(Ons)
  Iarm/1 -> MATLAB Function/4(Iarm)

== system Mmc_GFL_template/MMC/modulation/Sorting pa ==
  note: A secrect, unintelligible, confusing and insrutable function with \if inside \for inside \if inside \if inside \if
  Usm : Inport
  N : Inport  Port=2
  Iarm : Inport  Port=3
  Constant : Constant  Value=SigmaM
  Logical Operator : Logic  Operator=NOT  AllPortsSameDT=off  OutDataTypeStr=float('double')
  MATLAB Function : MATLAB Function  TreatAsAtomicUnit=on
  MATLAB Function1 : MATLAB Function  TreatAsAtomicUnit=on
  Memory : Memory  InitialCondition=logical(zeros(Nb_PM, 1))  InheritSampleTime=on
  Mux : Mux  Inputs=2
  firing : Outport
  wires:
  Iarm/1 -> MATLAB Function/4(Iarm)
  Memory/1 -> MATLAB Function/5(Ons)
  N/1 -> MATLAB Function/2(N)
  Constant/1 -> MATLAB Function/3(Sigmam)
  Usm/1 -> MATLAB Function/1(Usm)
  Mux/1 -> MATLAB Function1/1(u)
  MATLAB Function/1(Ons_next) -> Memory/1, Logical Operator/1, Mux/1
  Logical Operator/1 -> Mux/2
  MATLAB Function1/1(y) -> firing/1

== system Mmc_GFL_template/MMC/modulation/Sorting pb ==
  note: A secrect, unintelligible, confusing and insrutable function with \if inside \for inside \if inside \if inside \if
  Usm : Inport
  N : Inport  Port=2
  Iarm : Inport  Port=3
  Constant : Constant  Value=SigmaM
  Logical Operator : Logic  Operator=NOT  AllPortsSameDT=off  OutDataTypeStr=float('double')
  MATLAB Function : MATLAB Function  TreatAsAtomicUnit=on
  MATLAB Function1 : MATLAB Function  TreatAsAtomicUnit=on
  Memory : Memory  InitialCondition=logical(zeros(Nb_PM, 1))  InheritSampleTime=on
  Mux : Mux  Inputs=2
  firing : Outport
  wires:
  Iarm/1 -> MATLAB Function/4(Iarm)
  Memory/1 -> MATLAB Function/5(Ons)
  N/1 -> MATLAB Function/2(N)
  Constant/1 -> MATLAB Function/3(Sigmam)
  Usm/1 -> MATLAB Function/1(Usm)
  Mux/1 -> MATLAB Function1/1(u)
  MATLAB Function/1(Ons_next) -> Memory/1, Logical Operator/1, Mux/1
  Logical Operator/1 -> Mux/2
  MATLAB Function1/1(y) -> firing/1

== system Mmc_GFL_template/MMC/modulation/Sorting pb1 ==
  note: A secrect, unintelligible, confusing and insrutable function with \if inside \for inside \if inside \if inside \if
  Usm : Inport
  N : Inport  Port=2
  Iarm : Inport  Port=3
  Constant : Constant  Value=SigmaM
  Logical Operator : Logic  Operator=NOT  AllPortsSameDT=off  OutDataTypeStr=float('double')
  MATLAB Function : MATLAB Function  TreatAsAtomicUnit=on
  MATLAB Function1 : MATLAB Function  TreatAsAtomicUnit=on
  Memory : Memory  InitialCondition=logical(zeros(Nb_PM, 1))  InheritSampleTime=on
  Mux : Mux  Inputs=2
  firing : Outport
  wires:
  Iarm/1 -> MATLAB Function/4(Iarm)
  Memory/1 -> MATLAB Function/5(Ons)
  N/1 -> MATLAB Function/2(N)
  Constant/1 -> MATLAB Function/3(Sigmam)
  Usm/1 -> MATLAB Function/1(Usm)
  Mux/1 -> MATLAB Function1/1(u)
  MATLAB Function/1(Ons_next) -> Memory/1, Logical Operator/1, Mux/1
  Logical Operator/1 -> Mux/2
  MATLAB Function1/1(y) -> firing/1

== system Mmc_GFL_template/MMC/modulation/Sorting pc ==
  note: A secrect, unintelligible, confusing and insrutable function with \if inside \for inside \if inside \if inside \if
  Usm : Inport
  N : Inport  Port=2
  Iarm : Inport  Port=3
  Constant : Constant  Value=SigmaM
  Logical Operator : Logic  Operator=NOT  AllPortsSameDT=off  OutDataTypeStr=float('double')
  MATLAB Function : MATLAB Function  TreatAsAtomicUnit=on
  MATLAB Function1 : MATLAB Function  TreatAsAtomicUnit=on
  Memory : Memory  InitialCondition=logical(zeros(Nb_PM, 1))  InheritSampleTime=on
  Mux : Mux  Inputs=2
  firing : Outport
  wires:
  Iarm/1 -> MATLAB Function/4(Iarm)
  Memory/1 -> MATLAB Function/5(Ons)
  N/1 -> MATLAB Function/2(N)
  Constant/1 -> MATLAB Function/3(Sigmam)
  Usm/1 -> MATLAB Function/1(Usm)
  Mux/1 -> MATLAB Function1/1(u)
  MATLAB Function/1(Ons_next) -> Memory/1, Logical Operator/1, Mux/1
  Logical Operator/1 -> Mux/2
  MATLAB Function1/1(y) -> firing/1

== system Mmc_GFL_template/MMC/modulation/Subsystem1 ==
  ref : Inport
  PWM Generator (Multilevel) : eePwmGeneratorMultilevel/PWM Generator (Multilevel)  topology=Full-bridge  Nsm=Nb_PM  Tper=1/fs  Ts=Ts_Power
  Scope : Scope
  Upper arm a : MATLAB Function  TreatAsAtomicUnit=on
  n_pwm : Outport
  wires:
  PWM Generator (Multilevel)/1 -> Upper arm a/1(signals)
  Upper arm a/1(n_pwm) -> Scope/1, n_pwm/1
  ref/1 -> PWM Generator (Multilevel)/1

== system Mmc_GFL_template/MMC/modulation/Subsystem10 ==
  ref : Inport
  PWM Generator (Multilevel) : eePwmGeneratorMultilevel/PWM Generator (Multilevel)  topology=Full-bridge  Nsm=Nb_PM  Tper=1/fs  Ts=Ts_Power
  Scope : Scope
  Upper arm a : MATLAB Function  TreatAsAtomicUnit=on
  n_pwm : Outport
  wires:
  ref/1 -> PWM Generator (Multilevel)/1
  Upper arm a/1(n_pwm) -> n_pwm/1, Scope/1
  PWM Generator (Multilevel)/1 -> Upper arm a/1(signals)

== system Mmc_GFL_template/MMC/modulation/Subsystem11 ==
  ref : Inport
  PWM Generator (Multilevel) : eePwmGeneratorMultilevel/PWM Generator (Multilevel)  topology=Full-bridge  Nsm=Nb_PM  Tper=1/fs  Ts=Ts_Power
  Scope : Scope
  Upper arm a : MATLAB Function  TreatAsAtomicUnit=on
  n_pwm : Outport
  wires:
  PWM Generator (Multilevel)/1 -> Upper arm a/1(signals)
  Upper arm a/1(n_pwm) -> Scope/1, n_pwm/1
  ref/1 -> PWM Generator (Multilevel)/1

== system Mmc_GFL_template/MMC/modulation/Subsystem6 ==
  ref : Inport
  PWM Generator (Multilevel) : eePwmGeneratorMultilevel/PWM Generator (Multilevel)  topology=Half-bridge  Nsm=Nb_PM  Tper=1/fs  Ts=Ts_Power
  Scope : Scope
  Upper arm a : MATLAB Function  TreatAsAtomicUnit=on
  n_pwm : Outport
  wires:
  ref/1 -> PWM Generator (Multilevel)/1
  Upper arm a/1(n_pwm) -> n_pwm/1, Scope/1
  PWM Generator (Multilevel)/1 -> Upper arm a/1(signals)

== system Mmc_GFL_template/MMC/modulation/Subsystem7 ==
  ref : Inport
  PWM Generator (Multilevel) : eePwmGeneratorMultilevel/PWM Generator (Multilevel)  topology=Full-bridge  Nsm=Nb_PM  Tper=1/fs  Ts=Ts_Power
  Scope : Scope
  Upper arm a : MATLAB Function  TreatAsAtomicUnit=on
  n_pwm : Outport
  wires:
  PWM Generator (Multilevel)/1 -> Upper arm a/1(signals)
  Upper arm a/1(n_pwm) -> Scope/1, n_pwm/1
  ref/1 -> PWM Generator (Multilevel)/1

== system Mmc_GFL_template/MMC/modulation/Subsystem8 ==
  ref : Inport
  PWM Generator (Multilevel) : eePwmGeneratorMultilevel/PWM Generator (Multilevel)  topology=Full-bridge  Nsm=Nb_PM  Tper=1/fs  Ts=Ts_Power
  Scope : Scope
  Upper arm a : MATLAB Function  TreatAsAtomicUnit=on
  n_pwm : Outport
  wires:
  ref/1 -> PWM Generator (Multilevel)/1
  Upper arm a/1(n_pwm) -> n_pwm/1, Scope/1
  PWM Generator (Multilevel)/1 -> Upper arm a/1(signals)

== system Mmc_GFL_template/MMC/modulation/Subsystem9 ==
  ref : Inport
  PWM Generator (Multilevel) : eePwmGeneratorMultilevel/PWM Generator (Multilevel)  topology=Full-bridge  Nsm=Nb_PM  Tper=1/fs  Ts=Ts_Power
  Scope : Scope
  Upper arm a : MATLAB Function  TreatAsAtomicUnit=on
  n_pwm : Outport
  wires:
  PWM Generator (Multilevel)/1 -> Upper arm a/1(signals)
  Upper arm a/1(n_pwm) -> Scope/1, n_pwm/1
  ref/1 -> PWM Generator (Multilevel)/1

== matlab function Mmc_GFL_template/MMC/modulation/Sorting na/MATLAB Function1 ==
  data: u input; y output
function y = FiringSorting(u)
    y = u;
    for i = 1: length(u)
        if mod(i, 2) == 1
            y(i) = u(int16(i/2));
        else
            y(i) = u(int16(i/2+length(u)/2));
        end
    end
end

== matlab function Mmc_GFL_template/MMC/modulation/Sorting pb1/MATLAB Function ==
  data: Usm input; N input; Ons_next output; Sigmam input; Iarm input; Ons input
function Ons_next = SmFiringSorting(Usm, N, Sigmam, Iarm, Ons)
    %%%
    % SmFiringSorting -- SM firing sorting. -- C.SI on 5th, Oct.
    %% Inputs:
    % Usm - capacitor voltage on each SM;
    % N - number of SMs that needed to fire up;
    % Sigmam [%] - Maximum allowed voltage unbalance rate;
    % Iarm - arm current;
    % Ons (boolean) - indicate those SM(s) who are in series with the
    % source in the last control period;
    %% Outputs:
    % Ons_now (boolean) - indicate those SM(s) who should be in series with 
    % the source in this control period;
    %%%
    
    % number of SMs
    Nb = length(Usm);
    % initialize the on-state boolean array
    Ons_next = zeros(Nb, 1); 
    % rank the SMs in the order of descendance
    [~, order] = sort(Usm, 'descend');
    
    if max(abs(1-Usm)) > Sigmam/100
        % Over the maximum unbalance acceptance
        if Iarm > 0
            % charge the capacitors with lowest voltages
            Ons_next(order(Nb-N+1: Nb)) = ~Ons_next(order(Nb-N+1: Nb));
        else
            % discharge the capacitors with highest voltages
            Ons_next(order(1: N)) = ~Ons_next(order(1: N));
        end

    else
        if N-sum(Ons) ==  0
            % if we don't need to change the number of SM that is on
            Ons_next = Ons;
        
        elseif N-sum(Ons) > 0
            % if we need more SMs are to be on-state

            % number of SMs that needed to be changed the state
            DeltaN = N-sum(Ons);
            % keep previously being on SMs still being on
            Ons_next = Ons;

            if Iarm > 0
                % charge the capacitors with lowest voltages
                for i = 1: Nb
                    if DeltaN <= 0
                        break;
                    end
                    % if the SM is off and still need more SM
                    if Ons(order(Nb-i+1)) == false
                        DeltaN = DeltaN - 1;
                        Ons_next(order(Nb-i+1)) = true;
                    end
                end

            else
                % discharge the capacitors with highest voltages
                for i = 1: Nb
                    if DeltaN <= 0
                        break;
                    end
                    % if the SM is off and still need more SM
                    if Ons(order(i)) == false
                        DeltaN = DeltaN - 1;
                        Ons_next(order(i)) = true;
                    end
                end
            end

        else
            % if we need less SMs are to be on-state

            % number of SMs that needed to be changed the state
            DeltaN = sum(Ons)-N;
            % keep previously being on SMs still being on
            Ons_next = Ons;

            if Iarm > 0
                % remove the capacitor with highest voltage
                for i = 1: Nb
                    if DeltaN <= 0
                        break;
                    end
                    % if the SM is on and still need less SM
                    if Ons(order(i)) == true
                        DeltaN = DeltaN - 1;
                        Ons_next(order(i)) = false;
                    end
                end

            else
                % remove the capacitor with lowest voltage
                for i = 1: Nb
                    if DeltaN <= 0
                        break;
                    end
                    % if the SM is on and still need less SM
                    if Ons(order(Nb-i+1)) == true
                        DeltaN = DeltaN - 1;
                        Ons_next(order(Nb-i+1)) = false;
                    end
                end
            end
        end
    end
end
